simulink model "fboard_dwgn"  (Simulink 6.2)
settings: Solver=FixedStepDiscrete  SolverMode=SingleTasking  StartTime=0.0  StopTime=10.0  FixedStep=1  RelTol=1e-3
undefined symbols (not defined in the file): quant
libraries: xbsIndex_r3 x212, fb_xaui x1
(part 1 of 2)
settings Model: LastModifiedBy=mdexter
settings DebuggingCC: SolverPrmCheckMsg=warning

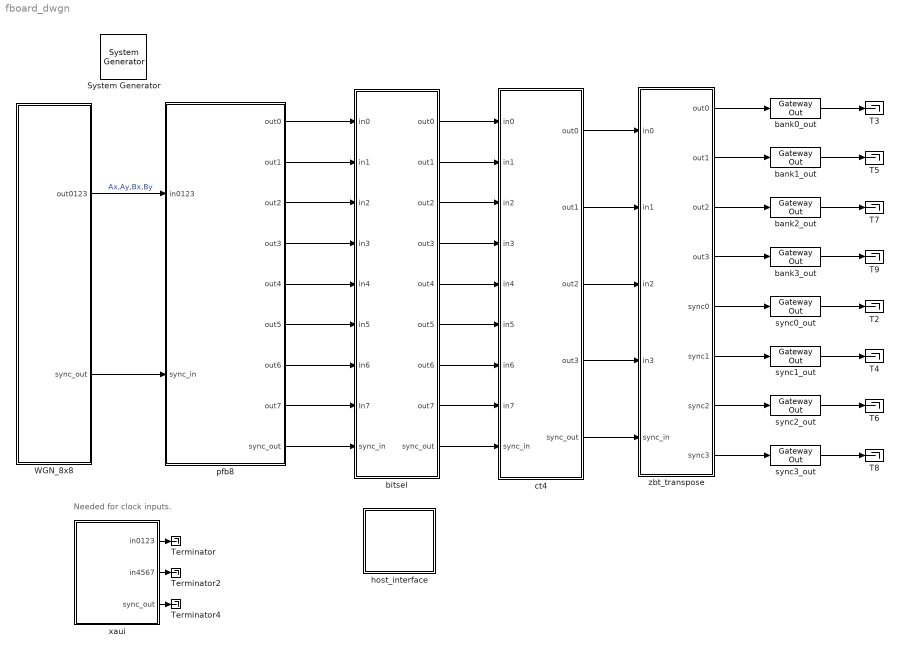
== system fboard_dwgn ==
  note: Needed for clock inputs.
  " System Generator" : xbsIndex_r3/ System Generator  Tag=genX  xilinxfamily=Virtex2P  part=xc2vp40  speed=-6  package=ff1152  synthesis_tool=XST  directory=./netlist  testbench=off  simulink_period=1  sysclk_period=100  incr_netlist=off  trim_vbits=Everywhere in SubSystem  dbl_ovrd=According to Block Masks  core_generation=According to Block Masks  run_coregen=off  deprecated_control=off  eval_field=0
      settings: AttributesFormatString=System\nGenerator
  T{2..9} (8 alike) : Terminator
  Terminator : Terminator
  Terminator2 : Terminator
  Terminator4 : Terminator
  WGN_8x8 : Subsystem
  bank0_out : xbsIndex_r3/Gateway Out  output_type=Double  nbits=8  bin_pt=6  arith_type=Boolean  quantization=Truncate  overflow=Wrap  hdl_port=on  timing_constraint=None  locs_specified=off  LOCs={}  needs_fixed_name=off  show_param=off
      settings: xl_area=[0, 0, 0, 0, 0, 0, 0]
  bank1_out : xbsIndex_r3/Gateway Out  output_type=Double  nbits=8  bin_pt=6  arith_type=Boolean  quantization=Truncate  overflow=Wrap  hdl_port=on  timing_constraint=None  locs_specified=off  LOCs={}  needs_fixed_name=off  show_param=off
      settings: xl_area=[0, 0, 0, 0, 0, 0, 0]
  bank2_out : xbsIndex_r3/Gateway Out  output_type=Double  nbits=8  bin_pt=6  arith_type=Boolean  quantization=Truncate  overflow=Wrap  hdl_port=on  timing_constraint=None  locs_specified=off  LOCs={}  needs_fixed_name=off  show_param=off
      settings: xl_area=[0, 0, 0, 0, 0, 0, 0]
  bank3_out : xbsIndex_r3/Gateway Out  output_type=Double  nbits=8  bin_pt=6  arith_type=Boolean  quantization=Truncate  overflow=Wrap  hdl_port=on  timing_constraint=None  locs_specified=off  LOCs={}  needs_fixed_name=off  show_param=off
      settings: xl_area=[0, 0, 0, 0, 0, 0, 0]
  bitsel : Subsystem
  ct4 : Subsystem
  host_interface : Subsystem
  pfb8 : Subsystem
  sync0_out : xbsIndex_r3/Gateway Out  output_type=Double  nbits=8  bin_pt=6  arith_type=Boolean  quantization=Truncate  overflow=Wrap  hdl_port=on  timing_constraint=None  locs_specified=off  LOCs={}  needs_fixed_name=off  show_param=off
      settings: xl_area=[0, 0, 0, 0, 0, 0, 0]
  sync1_out : xbsIndex_r3/Gateway Out  output_type=Double  nbits=8  bin_pt=6  arith_type=Boolean  quantization=Truncate  overflow=Wrap  hdl_port=on  timing_constraint=None  locs_specified=off  LOCs={}  needs_fixed_name=off  show_param=off
      settings: xl_area=[0, 0, 0, 0, 0, 0, 0]
  sync2_out : xbsIndex_r3/Gateway Out  output_type=Double  nbits=8  bin_pt=6  arith_type=Boolean  quantization=Truncate  overflow=Wrap  hdl_port=on  timing_constraint=None  locs_specified=off  LOCs={}  needs_fixed_name=off  show_param=off
      settings: xl_area=[0, 0, 0, 0, 0, 0, 0]
  sync3_out : xbsIndex_r3/Gateway Out  output_type=Double  nbits=8  bin_pt=6  arith_type=Boolean  quantization=Truncate  overflow=Wrap  hdl_port=on  timing_constraint=None  locs_specified=off  LOCs={}  needs_fixed_name=off  show_param=off
      settings: xl_area=[0, 0, 0, 0, 0, 0, 0]
  xaui : Subsystem
  zbt_transpose : Subsystem
  wires:
  WGN_8x8/1(out0123) -> pfb8/1(in0123)  "Ax,Ay,Bx,By"
  WGN_8x8/2(sync_out) -> pfb8/2(sync_in)
  sync0_out/1 -> T2/1
  bank0_out/1 -> T3/1
  sync1_out/1 -> T4/1
  bank1_out/1 -> T5/1
  sync2_out/1 -> T6/1
  bank2_out/1 -> T7/1
  sync3_out/1 -> T8/1
  bank3_out/1 -> T9/1
  pfb8/1(out0) -> bitsel/1(in0)
  pfb8/2(out1) -> bitsel/2(in1)
  pfb8/3(out2) -> bitsel/3(in2)
  pfb8/4(out3) -> bitsel/4(in3)
  pfb8/5(out4) -> bitsel/5(in4)
  pfb8/6(out5) -> bitsel/6(in5)
  pfb8/7(out6) -> bitsel/7(In6)
  pfb8/8(out7) -> bitsel/8(In7)
  pfb8/9(sync_out) -> bitsel/9(sync_in)
  bitsel/1(out0) -> ct4/1(in0)
  ct4/1(out0) -> zbt_transpose/1("in0\t")
  ct4/2(out1) -> zbt_transpose/2(in1)
  ct4/3(out2) -> zbt_transpose/3(in2)
  ct4/4(out3) -> zbt_transpose/4(in3)
  ct4/5(sync_out) -> zbt_transpose/5(sync_in)
  zbt_transpose/1(out0) -> bank0_out/1
  zbt_transpose/2(out1) -> bank1_out/1
  zbt_transpose/3(out2) -> bank2_out/1
  zbt_transpose/4(out3) -> bank3_out/1
  zbt_transpose/5(sync0) -> sync0_out/1
  zbt_transpose/6(sync1) -> sync1_out/1
  zbt_transpose/7(sync2) -> sync2_out/1
  zbt_transpose/8(sync3) -> sync3_out/1
  bitsel/2(out1) -> ct4/2(in1)
  bitsel/3(out2) -> ct4/3(in2)
  bitsel/4(out3) -> ct4/4(in3)
  bitsel/5(out4) -> ct4/5(in4)
  bitsel/6(out5) -> ct4/6(in5)
  bitsel/7(out6) -> ct4/7(in6)
  bitsel/8(out7) -> ct4/8(in7)
  bitsel/9(sync_out) -> ct4/9(sync_in)
  xaui/1(in0123) -> Terminator/1
  xaui/2(in4567) -> Terminator2/1
  xaui/3(sync_out) -> Terminator4/1

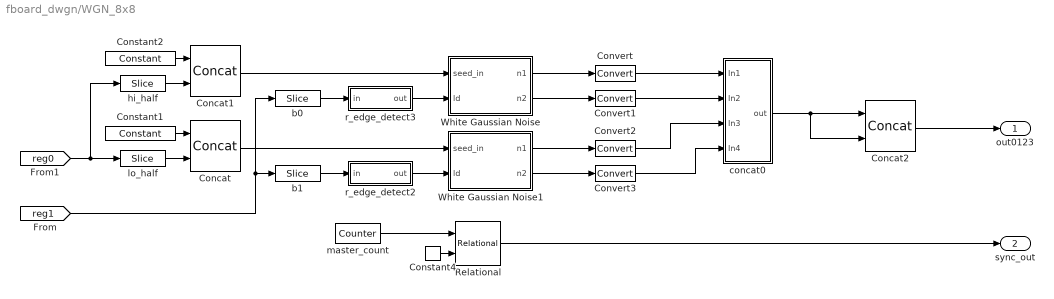
== system fboard_dwgn/WGN_8x8 ==
  Concat : xbsIndex_r3/Concat  num_inputs=2  explicit_period=off  period=1  dbl_ovrd=off
  Concat1 : xbsIndex_r3/Concat  num_inputs=2  explicit_period=off  period=1  dbl_ovrd=off
  Concat2 : xbsIndex_r3/Concat  num_inputs=2  explicit_period=off  period=1  dbl_ovrd=off
  Constant1 : xbsIndex_r3/Constant  const=hex2dec('bafd')  equ=P=C  arith_type=Unsigned  n_bits=16  bin_pt=0  opselect=C  inp2=PCIN>>17  opr=+  inp1=P  carry=CIN  iostate=0  explicit_period=on  period=1  dbl_ovrd=off
  Constant2 : xbsIndex_r3/Constant  const=hex2dec('bafd')  equ=P=C  arith_type=Unsigned  n_bits=16  bin_pt=0  opselect=C  inp2=PCIN>>17  opr=+  inp1=P  carry=CIN  iostate=0  explicit_period=on  period=1  dbl_ovrd=off
  Constant4 : xbsIndex_r3/Constant  const=0  equ=P=C  arith_type=Unsigned  n_bits=27  bin_pt=0  opselect=C  inp2=PCIN>>17  opr=+  inp1=P  carry=CIN  iostate=0  explicit_period=on  period=1  dbl_ovrd=off
  Convert{,1..3} (4 alike) : xbsIndex_r3/Convert  arith_type="Signed  (2's comp)"  n_bits=8  bin_pt=5  quantization="Round  (unbiased: +/- Inf)"  overflow=Wrap  latency=3  explicit_period=off  period=1  dbl_ovrd=off  show_param=on  inserted_by_tool=off  pipeline=on
      settings: xl_area=[0, 0, 0, 0, 0, 0, 0]
  Relational : xbsIndex_r3/Relational  mode=a=b  latency=1  explicit_period=off  period=1  en=off  dbl_ovrd=off  show_param=off
      settings: xl_area=[0, 0, 0, 0, 0, 0, 0]
  White Gaussian Noise : Subsystem  mask(Mask Type Goes Here){seed=hex2dec('12345678')}
      mask help: Mask Description Goes Here
      mask Help: Mask Help Goes Here
      mask CallbackString:
      | if str2num(get_param(gcb, 'seed')) == 0
      |     error('Seed cannot be zero.')
      | end
      mask Display:
      | port_label('input',1,'seed_in');
      | port_label('input',2,'ld');
      | port_label('output',1,'n1');
      | port_label('output',2,'n2');
  White Gaussian Noise1 : Subsystem  mask(Mask Type Goes Here){seed=hex2dec('12345678')}
      mask help: Mask Description Goes Here
      mask Help: Mask Help Goes Here
      mask CallbackString:
      | if str2num(get_param(gcb, 'seed')) == 0
      |     error('Seed cannot be zero.')
      | end
      mask Display:
      | port_label('input',1,'seed_in');
      | port_label('input',2,'ld');
      | port_label('output',1,'n1');
      | port_label('output',2,'n2');
  b0 : xbsIndex_r3/Slice  mode=Lower Bit Location + Width  nbits=1  bit1=0  base1=MSB of Input  bit0=0  base0=LSB of Input  boolean_output=on  explicit_period=off  period=1  dbl_ovrd=off
  b1 : xbsIndex_r3/Slice  mode=Lower Bit Location + Width  nbits=1  bit1=0  base1=MSB of Input  bit0=1  base0=LSB of Input  boolean_output=on  explicit_period=off  period=1  dbl_ovrd=off
  concat0 : Subsystem
  hi_half : xbsIndex_r3/Slice  mode=Upper Bit Location + Width  nbits=16  bit1=0  base1=MSB of Input  bit0=0  base0=LSB of Input  boolean_output=off  explicit_period=off  period=1  dbl_ovrd=off
  lo_half : xbsIndex_r3/Slice  mode=Lower Bit Location + Width  nbits=16  bit1=0  base1=MSB of Input  bit0=0  base0=LSB of Input  boolean_output=off  explicit_period=off  period=1  dbl_ovrd=off
  master_count : xbsIndex_r3/Counter  cnt_type=Free Running  n_bits=27  bin_pt=0  arith_type=Unsigned  start_count=0  cnt_to=Inf  cnt_by_val=1  operation=Up  explicit_period=off  period=1  load_pin=off  rst=off  en=off  dbl_ovrd=off  show_param=on  use_rpm=on  gen_core=off
      settings: xl_area=[0, 0, 0, 0, 0, 0, 0]
  r_edge_detect2 : Subsystem
  r_edge_detect3 : Subsystem
  out0123 : Outport
  sync_out : Outport  Port=2
  wires:
  White Gaussian Noise/1(n1) -> Convert/1
  White Gaussian Noise/2(n2) -> Convert1/1
  White Gaussian Noise1/1(n1) -> Convert2/1
  White Gaussian Noise1/2(n2) -> Convert3/1
  Convert/1 -> concat0/1(In1)
  Convert1/1 -> concat0/2(In2)
  Convert2/1 -> concat0/3(In3)
  Convert3/1 -> concat0/4(In4)
  concat0/1(out) -> Concat2/1, Concat2/2
  [reg1] -> b0/1, b1/1
  b0/1 -> r_edge_detect3/1(in)
  b1/1 -> r_edge_detect2/1(in)
  r_edge_detect2/1(out) -> White Gaussian Noise1/2(ld)
  r_edge_detect3/1(out) -> White Gaussian Noise/2(ld)
  master_count/1 -> Relational/1
  lo_half/1 -> Concat/2
  hi_half/1 -> Concat1/2
  Relational/1 -> sync_out/1
  [reg0] -> lo_half/1, hi_half/1
  Concat1/1 -> White Gaussian Noise/1(seed_in)
  Concat/1 -> White Gaussian Noise1/1(seed_in)
  Constant1/1 -> Concat/1
  Constant2/1 -> Concat1/1
  Constant4/1 -> Relational/2
  Concat2/1 -> out0123/1

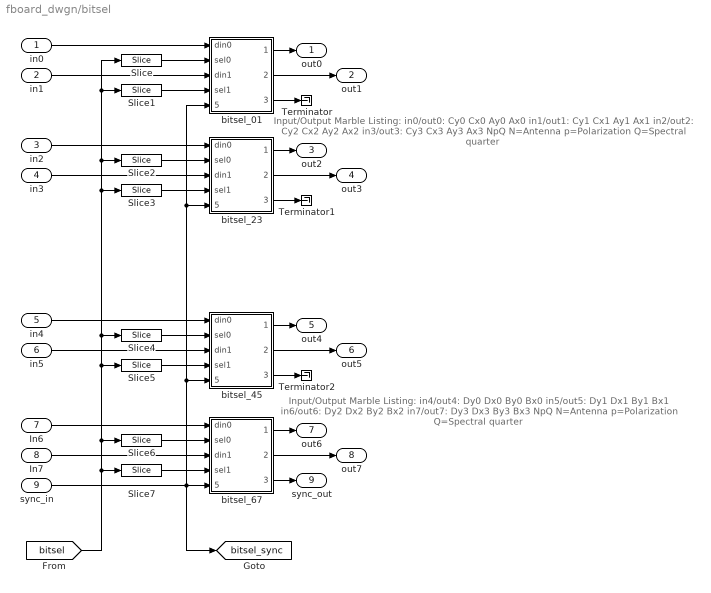
== system fboard_dwgn/bitsel ==
  note: Input/Output Marble Listing:
      |
      | in0/out0: Cy0 Cx0 Ay0 Ax0
      | in1/out1: Cy1 Cx1 Ay1 Ax1
      | in2/out2: Cy2 Cx2 Ay2 Ax2
      | in3/out3: Cy3 Cx3 Ay3 Ax3
      |
      | NpQ
      | N=Antenna
      | p=Polarization
      | Q=Spectral quarter
  note: Input/Output Marble Listing:
      |
      | in4/out4: Dy0 Dx0 By0 Bx0
      | in5/out5: Dy1 Dx1 By1 Bx1
      | in6/out6: Dy2 Dx2 By2 Bx2
      | in7/out7: Dy3 Dx3 By3 Bx3
      |
      | NpQ
      | N=Antenna
      | p=Polarization
      | Q=Spectral quarter
  in0 : Inport  Port=1  LatchInput=off
  in1 : Inport  Port=2  LatchInput=off
  in2 : Inport  Port=3  LatchInput=off
  in3 : Inport  Port=4  LatchInput=off
  in4 : Inport  Port=5  LatchInput=off
  in5 : Inport  Port=6  LatchInput=off
  In6 : Inport  Port=7  LatchInput=off
  In7 : Inport  Port=8  LatchInput=off
  sync_in : Inport  Port=9  LatchInput=off
  Slice : xbsIndex_r3/Slice  mode=Lower Bit Location + Width  nbits=4  bit1=0  base1=MSB of Input  bit0=0  base0=LSB of Input  boolean_output=off  explicit_period=off  period=1  dbl_ovrd=off
  Slice1 : xbsIndex_r3/Slice  mode=Lower Bit Location + Width  nbits=4  bit1=0  base1=MSB of Input  bit0=4  base0=LSB of Input  boolean_output=off  explicit_period=off  period=1  dbl_ovrd=off
  Slice2 : xbsIndex_r3/Slice  mode=Lower Bit Location + Width  nbits=4  bit1=0  base1=MSB of Input  bit0=8  base0=LSB of Input  boolean_output=off  explicit_period=off  period=1  dbl_ovrd=off
  Slice3 : xbsIndex_r3/Slice  mode=Lower Bit Location + Width  nbits=4  bit1=0  base1=MSB of Input  bit0=12  base0=LSB of Input  boolean_output=off  explicit_period=off  period=1  dbl_ovrd=off
  Slice4 : xbsIndex_r3/Slice  mode=Lower Bit Location + Width  nbits=4  bit1=0  base1=MSB of Input  bit0=16  base0=LSB of Input  boolean_output=off  explicit_period=off  period=1  dbl_ovrd=off
  Slice5 : xbsIndex_r3/Slice  mode=Lower Bit Location + Width  nbits=4  bit1=0  base1=MSB of Input  bit0=20  base0=LSB of Input  boolean_output=off  explicit_period=off  period=1  dbl_ovrd=off
  Slice6 : xbsIndex_r3/Slice  mode=Lower Bit Location + Width  nbits=4  bit1=0  base1=MSB of Input  bit0=24  base0=LSB of Input  boolean_output=off  explicit_period=off  period=1  dbl_ovrd=off
  Slice7 : xbsIndex_r3/Slice  mode=Lower Bit Location + Width  nbits=4  bit1=0  base1=MSB of Input  bit0=28  base0=LSB of Input  boolean_output=off  explicit_period=off  period=1  dbl_ovrd=off
  Terminator : Terminator
  Terminator1 : Terminator
  Terminator2 : Terminator
  bitsel_01 : Subsystem
  bitsel_23 : Subsystem
  bitsel_45 : Subsystem
  bitsel_67 : Subsystem
  out0 : Outport
  out1 : Outport  Port=2
  out2 : Outport  Port=3
  out3 : Outport  Port=4
  out4 : Outport  Port=5
  out5 : Outport  Port=6
  out6 : Outport  Port=7
  out7 : Outport  Port=8
  sync_out : Outport  Port=9
  tag scope: bitsel_sync=global
  wires:
  in0/1 -> bitsel_01/1(din0)
  bitsel_01/1(dout0) -> out0/1
  in1/1 -> bitsel_01/3(din1)
  in2/1 -> bitsel_23/1(din0)
  in3/1 -> bitsel_23/3(din1)
  in4/1 -> bitsel_45/1(din0)
  in5/1 -> bitsel_45/3(din1)
  In6/1 -> bitsel_67/1(din0)
  In7/1 -> bitsel_67/3(din1)
  sync_in/1 -> [bitsel_sync], bitsel_01/5(sync_in), bitsel_23/5(sync_in), bitsel_45/5(sync_in), bitsel_67/5(sync_in)
  Slice/1 -> bitsel_01/2(sel0)
  Slice1/1 -> bitsel_01/4(sel1)
  Slice2/1 -> bitsel_23/2(sel0)
  Slice3/1 -> bitsel_23/4(sel1)
  Slice4/1 -> bitsel_45/2(sel0)
  Slice5/1 -> bitsel_45/4(sel1)
  Slice6/1 -> bitsel_67/2(sel0)
  Slice7/1 -> bitsel_67/4(sel1)
  [bitsel] -> Slice5/1, Slice4/1, Slice3/1, Slice2/1, Slice1/1, Slice/1, Slice6/1, Slice7/1
  bitsel_01/3(sync_out) -> Terminator/1
  bitsel_01/2(dout1) -> out1/1
  bitsel_23/1(dout0) -> out2/1
  bitsel_23/3(sync_out) -> Terminator1/1
  bitsel_23/2(dout1) -> out3/1
  bitsel_45/1(dout0) -> out4/1
  bitsel_45/3(sync_out) -> Terminator2/1
  bitsel_45/2(dout1) -> out5/1
  bitsel_67/1(dout0) -> out6/1
  bitsel_67/2(dout1) -> out7/1
  bitsel_67/3(sync_out) -> sync_out/1

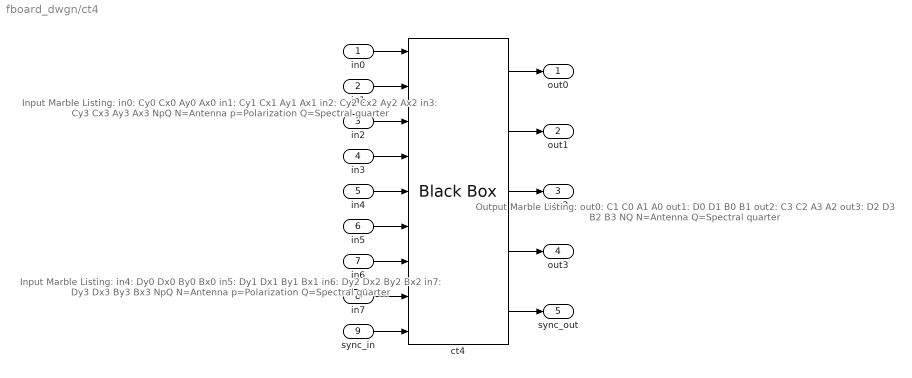
== system fboard_dwgn/ct4 ==
  note: Input Marble Listing:
      |
      | in0: Cy0 Cx0 Ay0 Ax0
      | in1: Cy1 Cx1 Ay1 Ax1
      | in2: Cy2 Cx2 Ay2 Ax2
      | in3: Cy3 Cx3 Ay3 Ax3
      |
      | NpQ
      | N=Antenna
      | p=Polarization
      | Q=Spectral quarter
  note: Input Marble Listing:
      |
      | in4: Dy0 Dx0 By0 Bx0
      | in5: Dy1 Dx1 By1 Bx1
      | in6: Dy2 Dx2 By2 Bx2
      | in7: Dy3 Dx3 By3 Bx3
      |
      | NpQ
      | N=Antenna
      | p=Polarization
      | Q=Spectral quarter
  note: Output Marble Listing:
      |
      | out0: C1 C0 A1 A0
      | out1: D0 D1 B0 B1
      | out2: C3 C2 A3 A2
      | out3: D2 D3 B2 B3
      |
      | NQ
      | N=Antenna
      | Q=Spectral quarter
  in0 : Inport  Port=1  LatchInput=off
  in1 : Inport  Port=2  LatchInput=off
  in2 : Inport  Port=3  LatchInput=off
  in3 : Inport  Port=4  LatchInput=off
  in4 : Inport  Port=5  LatchInput=off
  in5 : Inport  Port=6  LatchInput=off
  in6 : Inport  Port=7  LatchInput=off
  in7 : Inport  Port=8  LatchInput=off
  sync_in : Inport  Port=9  LatchInput=off
  ct4 : xbsIndex_r3/Black Box  init_code=ct4_config  sim_method=Inactive  show_param=off
      settings: xl_area=[0, 0, 0, 0, 0, 0, 0]
  out0 : Outport
  out1 : Outport  Port=2
  out2 : Outport  Port=3
  out3 : Outport  Port=4
  sync_out : Outport  Port=5
  wires:
  in0/1 -> ct4/1
  ct4/1 -> out0/1
  in1/1 -> ct4/2
  ct4/2 -> out1/1
  in2/1 -> ct4/3
  ct4/3 -> out2/1
  in3/1 -> ct4/4
  ct4/4 -> out3/1
  in4/1 -> ct4/5
  ct4/5 -> sync_out/1
  in5/1 -> ct4/6
  in6/1 -> ct4/7
  in7/1 -> ct4/8
  sync_in/1 -> ct4/9

== system fboard_dwgn/host_interface ==
  Constant2 : xbsIndex_r3/Constant  const=hex2dec('baff7ed')  equ=P=C  arith_type=Unsigned  n_bits=32  bin_pt=0  opselect=C  inp2=PCIN>>17  opr=+  inp1=P  carry=CIN  iostate=0  explicit_period=on  period=1  dbl_ovrd=off
  T12 : Terminator
  host_interface : xbsIndex_r3/Black Box  init_code=host_interface_config  sim_method=Inactive  show_param=off
      settings: xl_area=[0, 0, 0, 0, 0, 0, 0]
  reset : xbsIndex_r3/Gateway Out  output_type=Double  nbits=8  bin_pt=6  arith_type=Boolean  quantization=Truncate  overflow=Wrap  hdl_port=on  timing_constraint=None  locs_specified=off  LOCs={}  needs_fixed_name=off  show_param=off
      settings: xl_area=[0, 0, 0, 0, 0, 0, 0]
  tag scope: bitsel=global, reg0=global, reg1=global, reset=global
  wires:
  reset/1 -> T12/1
  [bitsel_sync] -> host_interface/1
  host_interface/4 -> reset/1, [reset]
  host_interface/1 -> [bitsel]
  host_interface/2 -> [reg0]
  host_interface/3 -> [reg1]
  Constant2/1 -> host_interface/2, host_interface/3, host_interface/4, host_interface/5, host_interface/6, host_interface/7, host_interface/8

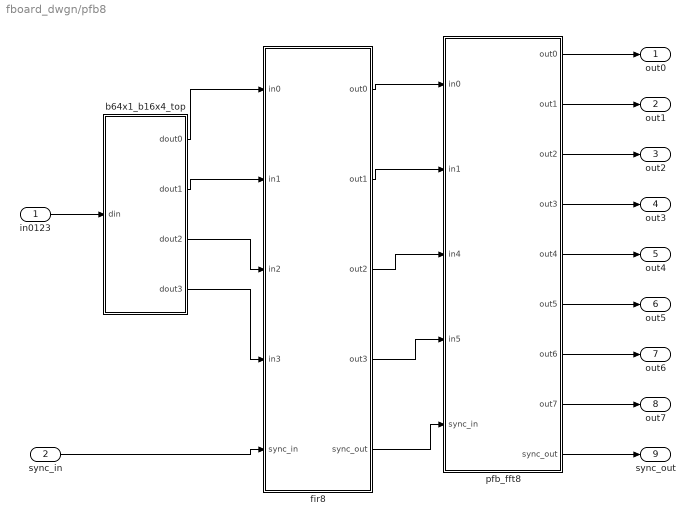
== system fboard_dwgn/pfb8 ==
  in0123 : Inport  Port=1  LatchInput=off
  sync_in : Inport  Port=2  LatchInput=off
  b64x1_b16x4_top : Subsystem
  fir8 : Subsystem  mask{fb_ntaps=4}
      mask prompts: fb_ntaps "Number of taps"
  pfb_fft8 : Subsystem
  out0 : Outport
  out1 : Outport  Port=2
  out2 : Outport  Port=3
  out3 : Outport  Port=4
  out4 : Outport  Port=5
  out5 : Outport  Port=6
  out6 : Outport  Port=7
  out7 : Outport  Port=8
  sync_out : Outport  Port=9
  wires:
  fir8/5(sync_out) -> pfb_fft8/5(sync_in)
  fir8/2(out1) -> pfb_fft8/2(in1)
  fir8/1(out0) -> pfb_fft8/1(in0)
  b64x1_b16x4_top/2(dout1) -> fir8/2(in1)
  b64x1_b16x4_top/1(dout0) -> fir8/1(in0)
  b64x1_b16x4_top/4(dout3) -> fir8/4(in3)
  b64x1_b16x4_top/3(dout2) -> fir8/3(in2)
  pfb_fft8/1(out0) -> out0/1
  pfb_fft8/2(out1) -> out1/1
  in0123/1 -> b64x1_b16x4_top/1(din)
  pfb_fft8/3(out2) -> out2/1
  pfb_fft8/4(out3) -> out3/1
  pfb_fft8/5(out4) -> out4/1
  pfb_fft8/6(out5) -> out5/1
  pfb_fft8/7(out6) -> out6/1
  pfb_fft8/8(out7) -> out7/1
  pfb_fft8/9(sync_out) -> sync_out/1
  sync_in/1 -> fir8/5(sync_in)
  fir8/3(out2) -> pfb_fft8/3(in4)
  fir8/4(out3) -> pfb_fft8/4(in5)

== system fboard_dwgn/xaui ==
  Constant : xbsIndex_r3/Constant  const=0  equ=P=C  arith_type=Boolean  n_bits=1  bin_pt=0  opselect=C  inp2=PCIN>>17  opr=+  inp1=P  carry=CIN  iostate=0  explicit_period=on  period=1  dbl_ovrd=off
  Constant1 : xbsIndex_r3/Constant  const=1  equ=P=C  arith_type=Boolean  n_bits=1  bin_pt=0  opselect=C  inp2=PCIN>>17  opr=+  inp1=P  carry=CIN  iostate=0  explicit_period=on  period=1  dbl_ovrd=off
  Slice : xbsIndex_r3/Slice  mode=Lower Bit Location + Width  nbits=1  bit1=0  base1=MSB of Input  bit0=0  base0=LSB of Input  boolean_output=on  explicit_period=off  period=1  dbl_ovrd=off
  Slice1 : xbsIndex_r3/Slice  mode=Lower Bit Location + Width  nbits=1  bit1=0  base1=MSB of Input  bit0=0  base0=LSB of Input  boolean_output=on  explicit_period=off  period=1  dbl_ovrd=off
  fb_xaui : fb_xaui/fb_xaui
  realign : Subsystem
  status_monitor : Subsystem
  sync_monitor : Subsystem
  sync_sel : Subsystem
  in0123 : Outport
  in4567 : Outport  Port=2
  sync_out : Outport  Port=3
  wires:
  Constant/1 -> fb_xaui/1
  Constant1/1 -> fb_xaui/2
  fb_xaui/6 -> status_monitor/2(bot_status)
  fb_xaui/3 -> status_monitor/1(top_status)
  fb_xaui/1 -> realign/1(din0)
  fb_xaui/2 -> Slice/1
  fb_xaui/4 -> realign/3(din1)
  fb_xaui/5 -> Slice1/1
  Slice/1 -> sync_monitor/1(top_sync), realign/2(sync0), sync_sel/1(top_sync)
  Slice1/1 -> sync_monitor/2(bot_sync), realign/4(sync1), sync_sel/2(bot_sync)
  realign/1(dout0) -> in0123/1
  realign/2(dout1) -> in4567/1
  realign/3(sync_out) -> sync_out/1
  sync_sel/1(sync_out) -> realign/5(sync_in)

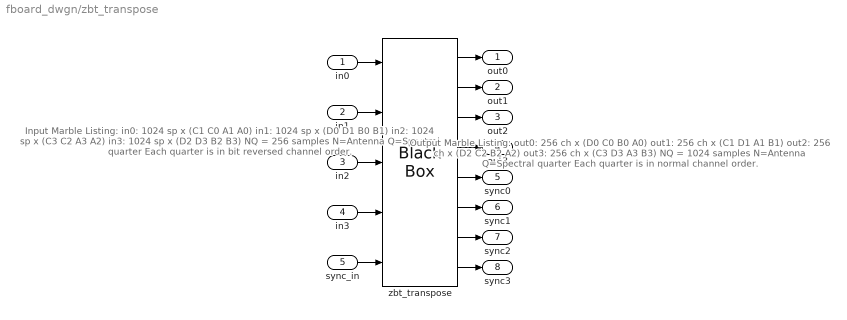
== system fboard_dwgn/zbt_transpose ==
  note: Input Marble Listing:
      |
      | in0: 1024 sp x (C1 C0 A1 A0)
      | in1: 1024 sp x (D0 D1 B0 B1)
      | in2: 1024 sp x (C3 C2 A3 A2)
      | in3: 1024 sp x (D2 D3 B2 B3)
      |
      | NQ = 256 samples
      |
      | N=Antenna
      | Q=Spectral quarter
      |
      | Each quarter is in bit
      | reversed channel order.
  note: Output Marble Listing:
      |
      | out0: 256 ch x (D0 C0 B0 A0)
      | out1: 256 ch x (C1 D1 A1 B1)
      | out2: 256 ch x (D2 C2 B2 A2)
      | out3: 256 ch x (C3 D3 A3 B3)
      |
      | NQ = 1024 samples
      |
      | N=Antenna
      | Q=Spectral quarter
      |
      | Each quarter is in
      | normal channel order.
  "in0\t" : Inport  Port=1  LatchInput=off
  in1 : Inport  Port=2  LatchInput=off
  in2 : Inport  Port=3  LatchInput=off
  in3 : Inport  Port=4  LatchInput=off
  sync_in : Inport  Port=5  LatchInput=off
  zbt_transpose : xbsIndex_r3/Black Box  init_code=zbt_transpose_config  sim_method=Inactive  show_param=off
      settings: xl_area=[0, 0, 0, 0, 0, 0, 0]
  out0 : Outport
  out1 : Outport  Port=2
  out2 : Outport  Port=3
  out3 : Outport  Port=4
  sync0 : Outport  Port=5
  sync1 : Outport  Port=6
  sync2 : Outport  Port=7
  sync3 : Outport  Port=8
  wires:
  zbt_transpose/1 -> out0/1
  "in0\t"/1 -> zbt_transpose/1
  zbt_transpose/2 -> out1/1
  in1/1 -> zbt_transpose/2
  zbt_transpose/3 -> out2/1
  zbt_transpose/4 -> out3/1
  in2/1 -> zbt_transpose/3
  zbt_transpose/5 -> sync0/1
  in3/1 -> zbt_transpose/4
  zbt_transpose/6 -> sync1/1
  zbt_transpose/7 -> sync2/1
  sync_in/1 -> zbt_transpose/5
  zbt_transpose/8 -> sync3/1

== system fboard_dwgn/WGN_8x8/White Gaussian Noise ==
  seed_in : Inport  Port=1  LatchInput=off
  ld : Inport  Port=2  LatchInput=off
  tt800_prng : Subsystem
  tt800_seed_gen : Subsystem
  u2n : Subsystem
  n1 : Outport
  n2 : Outport  Port=2
  wires:
  tt800_prng/1(out) -> u2n/1(u)
  tt800_seed_gen/1(seed_out) -> tt800_prng/1(seed)
  tt800_seed_gen/2(seed_en) -> tt800_prng/2(seed_en)
  seed_in/1 -> tt800_seed_gen/1(seed_in)
  u2n/1(n1) -> n1/1
  ld/1 -> tt800_seed_gen/2(ld)
  u2n/2(n2) -> n2/1

== system fboard_dwgn/WGN_8x8/White Gaussian Noise1 ==
  seed_in : Inport  Port=1  LatchInput=off
  ld : Inport  Port=2  LatchInput=off
  tt800_prng : Subsystem
  tt800_seed_gen : Subsystem
  u2n : Subsystem
  n1 : Outport
  n2 : Outport  Port=2
  wires:
  tt800_prng/1(out) -> u2n/1(u)
  tt800_seed_gen/1(seed_out) -> tt800_prng/1(seed)
  tt800_seed_gen/2(seed_en) -> tt800_prng/2(seed_en)
  seed_in/1 -> tt800_seed_gen/1(seed_in)
  u2n/1(n1) -> n1/1
  ld/1 -> tt800_seed_gen/2(ld)
  u2n/2(n2) -> n2/1

== system fboard_dwgn/WGN_8x8/concat0 ==
  In1 : Inport  Port=1  LatchInput=off
  In2 : Inport  Port=2  LatchInput=off
  In3 : Inport  Port=3  LatchInput=off
  In4 : Inport  Port=4  LatchInput=off
  ri_to_c : Subsystem  mask(Real-Imag to Complex){}
      mask help: Concatenates real and imaginary inputs into a complex output.
      mask init:
      | ri_to_c_init(gcb);
      mask Help:
      | <pre>
      | Description::
      | 
      | Concatenates a real and imaginary input into a complex output.
      | Useful for simplifying interconnects.
      | See also: Complex to Real-Imag (c_to_ri)
      | 
      | Mask Parameters::
      | 
      | (N/A)
      | </pre>
  ri_to_c1 : Subsystem  mask(Real-Imag to Complex){}
      mask help: Concatenates real and imaginary inputs into a complex output.
      mask init:
      | ri_to_c_init(gcb);
      mask Help:
      | <pre>
      | Description::
      | 
      | Concatenates a real and imaginary input into a complex output.
      | Useful for simplifying interconnects.
      | See also: Complex to Real-Imag (c_to_ri)
      | 
      | Mask Parameters::
      | 
      | (N/A)
      | </pre>
  ri_to_c2 : Subsystem  mask(Real-Imag to Complex){}
      mask help: Concatenates real and imaginary inputs into a complex output.
      mask init:
      | ri_to_c_init(gcb);
      mask Help:
      | <pre>
      | Description::
      | 
      | Concatenates a real and imaginary input into a complex output.
      | Useful for simplifying interconnects.
      | See also: Complex to Real-Imag (c_to_ri)
      | 
      | Mask Parameters::
      | 
      | (N/A)
      | </pre>
  out : Outport
  wires:
  ri_to_c/1(c) -> ri_to_c2/1(re)
  ri_to_c1/1(c) -> ri_to_c2/2(im)
  In1/1 -> ri_to_c/1(re)
  In2/1 -> ri_to_c/2(im)
  ri_to_c2/1(c) -> out/1
  In3/1 -> ri_to_c1/1(re)
  In4/1 -> ri_to_c1/2(im)

== system fboard_dwgn/WGN_8x8/r_edge_detect2 ==
  in : Inport  Port=1  LatchInput=off
  Delay : xbsIndex_r3/Delay  latency=1  reg_retiming=off  explicit_period=off  period=1  en=off  accept_only_valid=off  init_zero=on  dbl_ovrd=off  show_param=off
      settings: xl_area=[1 1 0 0 0 0 0]
  Expression : xbsIndex_r3/Expression  expression=curr & ~prev  precision=Full  arith_type=Unsigned  n_bits=8  bin_pt=2  align_bp=on  latency=0  explicit_period=off  period=1  en=off  dbl_ovrd=off  show_param=off
      settings: xl_area=[0, 0, 0, 0, 0, 0, 0]
  out : Outport
  wires:
  in/1 -> Expression/1, Delay/1
  Delay/1 -> Expression/2
  Expression/1 -> out/1

== system fboard_dwgn/WGN_8x8/r_edge_detect3 ==
  in : Inport  Port=1  LatchInput=off
  Delay : xbsIndex_r3/Delay  latency=1  reg_retiming=off  explicit_period=off  period=1  en=off  accept_only_valid=off  init_zero=on  dbl_ovrd=off  show_param=off
      settings: xl_area=[1 1 0 0 0 0 0]
  Expression : xbsIndex_r3/Expression  expression=curr & ~prev  precision=Full  arith_type=Unsigned  n_bits=8  bin_pt=2  align_bp=on  latency=0  explicit_period=off  period=1  en=off  dbl_ovrd=off  show_param=off
      settings: xl_area=[0, 0, 0, 0, 0, 0, 0]
  out : Outport
  wires:
  Expression/1 -> out/1
  Delay/1 -> Expression/2
  in/1 -> Delay/1, Expression/1

== system fboard_dwgn/bitsel/bitsel_01 ==
  note: If bitsel black box is too expensive,
      | use fixed bit selection via
      | complex_convert with 19_8 in.
  din0 : Inport  Port=1  LatchInput=off
  sel0 : Inport  Port=2  LatchInput=off
  din1 : Inport  Port=3  LatchInput=off
  sel1 : Inport  Port=4  LatchInput=off
  sync_in : Inport  Port=5  LatchInput=off
  Constant : xbsIndex_r3/Constant  const=0  equ=P=C  arith_type=Boolean  n_bits=1  bin_pt=0  opselect=C  inp2=PCIN>>17  opr=+  inp1=P  carry=CIN  iostate=0  explicit_period=on  period=1  dbl_ovrd=off
  Terminator : Terminator
  bitsel_0 : xbsIndex_r3/Black Box  init_code=bitsel_config  sim_method=Inactive  show_param=off
      settings: xl_area=[0, 0, 0, 0, 0, 0, 0]
  bitsel_1 : xbsIndex_r3/Black Box  init_code=bitsel_config  sim_method=Inactive  show_param=off
      settings: xl_area=[0, 0, 0, 0, 0, 0, 0]
  dout0 : Outport
  dout1 : Outport  Port=2
  sync_out : Outport  Port=3
  wires:
  din0/1 -> bitsel_0/1
  din1/1 -> bitsel_1/1
  sel0/1 -> bitsel_0/2
  bitsel_0/1 -> dout0/1
  sel1/1 -> bitsel_1/2
  bitsel_1/1 -> dout1/1
  sync_in/1 -> bitsel_1/3
  bitsel_1/2 -> sync_out/1
  Constant/1 -> bitsel_0/3
  bitsel_0/2 -> Terminator/1

== system fboard_dwgn/bitsel/bitsel_23 ==
  note: If bitsel black box is too expensive,
      | use fixed bit selection via
      | complex_convert with 19_8 in.
  din0 : Inport  Port=1  LatchInput=off
  sel0 : Inport  Port=2  LatchInput=off
  din1 : Inport  Port=3  LatchInput=off
  sel1 : Inport  Port=4  LatchInput=off
  sync_in : Inport  Port=5  LatchInput=off
  Constant : xbsIndex_r3/Constant  const=0  equ=P=C  arith_type=Boolean  n_bits=1  bin_pt=0  opselect=C  inp2=PCIN>>17  opr=+  inp1=P  carry=CIN  iostate=0  explicit_period=on  period=1  dbl_ovrd=off
  Terminator : Terminator
  bitsel_0 : xbsIndex_r3/Black Box  init_code=bitsel_config  sim_method=Inactive  show_param=off
      settings: xl_area=[0, 0, 0, 0, 0, 0, 0]
  bitsel_1 : xbsIndex_r3/Black Box  init_code=bitsel_config  sim_method=Inactive  show_param=off
      settings: xl_area=[0, 0, 0, 0, 0, 0, 0]
  dout0 : Outport
  dout1 : Outport  Port=2
  sync_out : Outport  Port=3
  wires:
  bitsel_0/2 -> Terminator/1
  Constant/1 -> bitsel_0/3
  bitsel_1/2 -> sync_out/1
  sync_in/1 -> bitsel_1/3
  bitsel_1/1 -> dout1/1
  sel1/1 -> bitsel_1/2
  bitsel_0/1 -> dout0/1
  sel0/1 -> bitsel_0/2
  din1/1 -> bitsel_1/1
  din0/1 -> bitsel_0/1

== system fboard_dwgn/bitsel/bitsel_45 ==
  note: If bitsel black box is too expensive,
      | use fixed bit selection via
      | complex_convert with 19_8 in.
  din0 : Inport  Port=1  LatchInput=off
  sel0 : Inport  Port=2  LatchInput=off
  din1 : Inport  Port=3  LatchInput=off
  sel1 : Inport  Port=4  LatchInput=off
  sync_in : Inport  Port=5  LatchInput=off
  Constant : xbsIndex_r3/Constant  const=0  equ=P=C  arith_type=Boolean  n_bits=1  bin_pt=0  opselect=C  inp2=PCIN>>17  opr=+  inp1=P  carry=CIN  iostate=0  explicit_period=on  period=1  dbl_ovrd=off
  Terminator : Terminator
  bitsel_0 : xbsIndex_r3/Black Box  init_code=bitsel_config  sim_method=Inactive  show_param=off
      settings: xl_area=[0, 0, 0, 0, 0, 0, 0]
  bitsel_1 : xbsIndex_r3/Black Box  init_code=bitsel_config  sim_method=Inactive  show_param=off
      settings: xl_area=[0, 0, 0, 0, 0, 0, 0]
  dout0 : Outport
  dout1 : Outport  Port=2
  sync_out : Outport  Port=3
  wires:
  din0/1 -> bitsel_0/1
  din1/1 -> bitsel_1/1
  sel0/1 -> bitsel_0/2
  bitsel_0/1 -> dout0/1
  sel1/1 -> bitsel_1/2
  bitsel_1/1 -> dout1/1
  sync_in/1 -> bitsel_1/3
  bitsel_1/2 -> sync_out/1
  Constant/1 -> bitsel_0/3
  bitsel_0/2 -> Terminator/1

== system fboard_dwgn/bitsel/bitsel_67 ==
  note: If bitsel black box is too expensive,
      | use fixed bit selection via
      | complex_convert with 19_8 in.
  din0 : Inport  Port=1  LatchInput=off
  sel0 : Inport  Port=2  LatchInput=off
  din1 : Inport  Port=3  LatchInput=off
  sel1 : Inport  Port=4  LatchInput=off
  sync_in : Inport  Port=5  LatchInput=off
  Constant : xbsIndex_r3/Constant  const=0  equ=P=C  arith_type=Boolean  n_bits=1  bin_pt=0  opselect=C  inp2=PCIN>>17  opr=+  inp1=P  carry=CIN  iostate=0  explicit_period=on  period=1  dbl_ovrd=off
  Terminator : Terminator
  bitsel_0 : xbsIndex_r3/Black Box  init_code=bitsel_config  sim_method=Inactive  show_param=off
      settings: xl_area=[0, 0, 0, 0, 0, 0, 0]
  bitsel_1 : xbsIndex_r3/Black Box  init_code=bitsel_config  sim_method=Inactive  show_param=off
      settings: xl_area=[0, 0, 0, 0, 0, 0, 0]
  dout0 : Outport
  dout1 : Outport  Port=2
  sync_out : Outport  Port=3
  wires:
  bitsel_0/2 -> Terminator/1
  Constant/1 -> bitsel_0/3
  bitsel_1/2 -> sync_out/1
  sync_in/1 -> bitsel_1/3
  bitsel_1/1 -> dout1/1
  sel1/1 -> bitsel_1/2
  bitsel_0/1 -> dout0/1
  sel0/1 -> bitsel_0/2
  din1/1 -> bitsel_1/1
  din0/1 -> bitsel_0/1

== system fboard_dwgn/pfb8/b64x1_b16x4_top ==
  din : Inport  Port=1  LatchInput=off
  Slice0 : xbsIndex_r3/Slice  mode=Lower Bit Location + Width  nbits=16  bit1=0  base1=LSB of Input  bit0=0  base0=LSB of Input  boolean_output=off  explicit_period=off  period=1  dbl_ovrd=off
  Slice1 : xbsIndex_r3/Slice  mode=Lower Bit Location + Width  nbits=16  bit1=0  base1=LSB of Input  bit0=16  base0=LSB of Input  boolean_output=off  explicit_period=off  period=1  dbl_ovrd=off
  Slice2 : xbsIndex_r3/Slice  mode=Lower Bit Location + Width  nbits=16  bit1=0  base1=LSB of Input  bit0=32  base0=LSB of Input  boolean_output=off  explicit_period=off  period=1  dbl_ovrd=off
  Slice3 : xbsIndex_r3/Slice  mode=Lower Bit Location + Width  nbits=16  bit1=0  base1=LSB of Input  bit0=48  base0=LSB of Input  boolean_output=off  explicit_period=off  period=1  dbl_ovrd=off
  dout0 : Outport
  dout1 : Outport  Port=2
  dout2 : Outport  Port=3
  dout3 : Outport  Port=4
  wires:
  din/1 -> Slice3/1, Slice2/1, Slice0/1, Slice1/1
  Slice3/1 -> dout0/1
  Slice2/1 -> dout1/1
  Slice1/1 -> dout2/1
  Slice0/1 -> dout3/1

== system fboard_dwgn/pfb8/fir8 ==
  in0 : Inport  Port=1  LatchInput=off
  in1 : Inport  Port=2  LatchInput=off
  in2 : Inport  Port=3  LatchInput=off
  in3 : Inport  Port=4  LatchInput=off
  sync_in : Inport  Port=5  LatchInput=off
  Terminator : Terminator
  pfb_fir_0 : Subsystem
  pfb_fir_1 : Subsystem
  out0 : Outport
  out1 : Outport  Port=2
  out2 : Outport  Port=3
  out3 : Outport  Port=4
  sync_out : Outport  Port=5
  wires:
  in0/1 -> pfb_fir_0/1(pol1_in)
  pfb_fir_0/1(pol1_out) -> out0/1
  in1/1 -> pfb_fir_0/2(pol2_in)
  pfb_fir_0/2(pol2_out) -> out1/1
  in2/1 -> pfb_fir_1/1(pol1_in)
  pfb_fir_1/1(pol1_out) -> out2/1
  in3/1 -> pfb_fir_1/2(pol2_in)
  pfb_fir_1/2(pol2_out) -> out3/1
  sync_in/1 -> pfb_fir_1/3(sync_in), pfb_fir_0/3(sync_in)
  pfb_fir_0/3(sync_out) -> Terminator/1
  pfb_fir_1/3(sync_out) -> sync_out/1

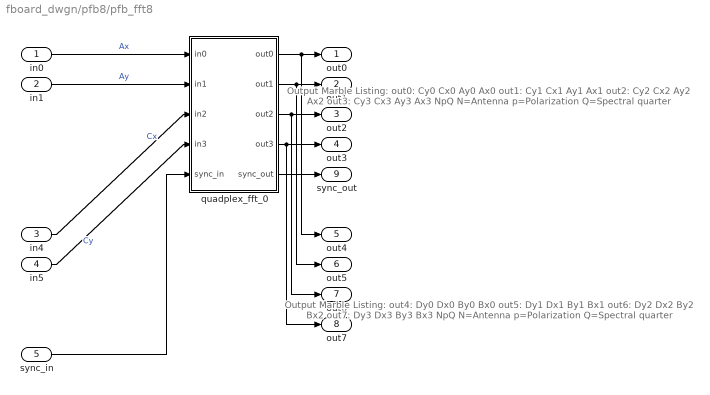
== system fboard_dwgn/pfb8/pfb_fft8 ==
  note: Output Marble Listing:
      |
      | out0: Cy0 Cx0 Ay0 Ax0
      | out1: Cy1 Cx1 Ay1 Ax1
      | out2: Cy2 Cx2 Ay2 Ax2
      | out3: Cy3 Cx3 Ay3 Ax3
      |
      | NpQ
      | N=Antenna
      | p=Polarization
      | Q=Spectral quarter
  note: Output Marble Listing:
      |
      | out4: Dy0 Dx0 By0 Bx0
      | out5: Dy1 Dx1 By1 Bx1
      | out6: Dy2 Dx2 By2 Bx2
      | out7: Dy3 Dx3 By3 Bx3
      |
      | NpQ
      | N=Antenna
      | p=Polarization
      | Q=Spectral quarter
  in0 : Inport  Port=1  LatchInput=off
  in1 : Inport  Port=2  LatchInput=off
  in4 : Inport  Port=3  LatchInput=off
  in5 : Inport  Port=4  LatchInput=off
  sync_in : Inport  Port=5  LatchInput=off
  quadplex_fft_0 : Subsystem
  out0 : Outport
  out1 : Outport  Port=2
  out2 : Outport  Port=3
  out3 : Outport  Port=4
  out4 : Outport  Port=5
  out5 : Outport  Port=6
  out6 : Outport  Port=7
  out7 : Outport  Port=8
  sync_out : Outport  Port=9
  wires:
  in0/1 -> quadplex_fft_0/1(in0)  "Ax"
  quadplex_fft_0/1(out0) -> out0/1, out4/1
  in1/1 -> quadplex_fft_0/2(in1)  "Ay"
  quadplex_fft_0/2(out1) -> out1/1, out5/1
  quadplex_fft_0/3(out2) -> out2/1, out6/1
  quadplex_fft_0/4(out3) -> out3/1, out7/1
  sync_in/1 -> quadplex_fft_0/5(sync_in)
  quadplex_fft_0/5(sync_out) -> sync_out/1
  in4/1 -> quadplex_fft_0/3(in2)  "Cx"
  in5/1 -> quadplex_fft_0/4(in3)  "Cy"

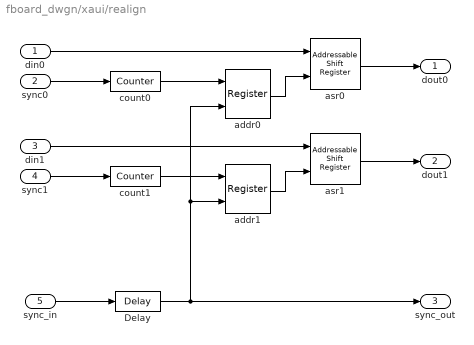
== system fboard_dwgn/xaui/realign ==
  din0 : Inport  Port=1  LatchInput=off
  sync0 : Inport  Port=2  LatchInput=off
  din1 : Inport  Port=3  LatchInput=off
  sync1 : Inport  Port=4  LatchInput=off
  sync_in : Inport  Port=5  LatchInput=off
  Delay : xbsIndex_r3/Delay  latency=1  reg_retiming=off  explicit_period=off  period=1  en=off  accept_only_valid=off  init_zero=on  dbl_ovrd=off  show_param=off
      settings: xl_area=[1 1 0 0 0 0 0]
  addr0 : xbsIndex_r3/Register  init=0  reg_only_valid=off  explicit_period=off  period=1  rst=off  en=on  out_en=off  dbl_ovrd=off  show_param=on
      settings: xl_area=[3 6 0 0 0 0 0]
  addr1 : xbsIndex_r3/Register  init=0  reg_only_valid=off  explicit_period=off  period=1  rst=off  en=on  out_en=off  dbl_ovrd=off  show_param=on
      settings: xl_area=[3 6 0 0 0 0 0]
  asr0 : xbsIndex_r3/Addressable Shift Register  infer_latency=on  depth=2  initVector=[0]  explicit_period=off  period=1  accept_only_valid=off  en=off  dbl_ovrd=off  show_param=on  use_rpm=on  gen_core=off
      settings: xl_area=[192 0 0 384 0 0 0]
  asr1 : xbsIndex_r3/Addressable Shift Register  infer_latency=on  depth=2  initVector=[0]  explicit_period=off  period=1  accept_only_valid=off  en=off  dbl_ovrd=off  show_param=on  use_rpm=on  gen_core=off
      settings: xl_area=[192 0 0 384 0 0 0]
  count0 : xbsIndex_r3/Counter  cnt_type=Free Running  n_bits=6  bin_pt=0  arith_type=Unsigned  start_count=0  cnt_to=Inf  cnt_by_val=1  operation=Up  explicit_period=off  period=1  load_pin=off  rst=on  en=off  dbl_ovrd=off  show_param=on  use_rpm=on  gen_core=off
      settings: xl_area=[3 6 0 6 0 0 0]
  count1 : xbsIndex_r3/Counter  cnt_type=Free Running  n_bits=6  bin_pt=0  arith_type=Unsigned  start_count=0  cnt_to=Inf  cnt_by_val=1  operation=Up  explicit_period=off  period=1  load_pin=off  rst=on  en=off  dbl_ovrd=off  show_param=on  use_rpm=on  gen_core=off
      settings: xl_area=[3 6 0 6 0 0 0]
  dout0 : Outport
  dout1 : Outport  Port=2
  sync_out : Outport  Port=3
  wires:
  count0/1 -> addr0/1
  addr0/1 -> asr0/2
  count1/1 -> addr1/1
  addr1/1 -> asr1/2
  Delay/1 -> addr1/2, addr0/2, sync_out/1
  din0/1 -> asr0/1
  asr0/1 -> dout0/1
  sync0/1 -> count0/1
  din1/1 -> asr1/1
  asr1/1 -> dout1/1
  sync1/1 -> count1/1
  sync_in/1 -> Delay/1

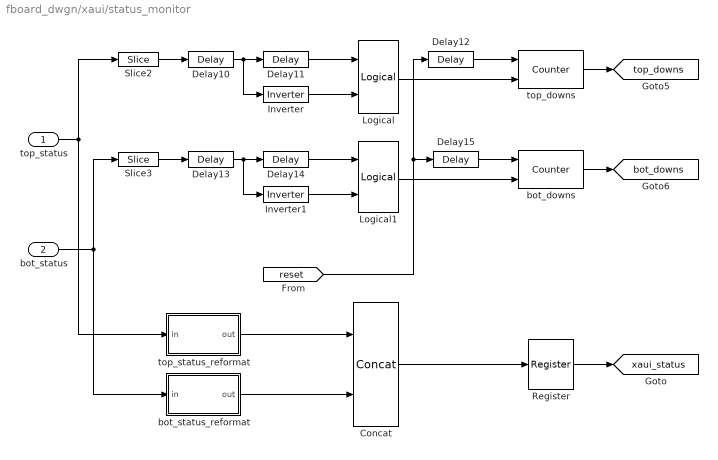
== system fboard_dwgn/xaui/status_monitor ==
  top_status : Inport  Port=1  LatchInput=off
  bot_status : Inport  Port=2  LatchInput=off
  Concat : xbsIndex_r3/Concat  num_inputs=2  explicit_period=off  period=1  dbl_ovrd=off
  Delay{10..15} (6 alike) : xbsIndex_r3/Delay  latency=1  reg_retiming=off  explicit_period=off  period=1  en=off  accept_only_valid=off  init_zero=on  dbl_ovrd=off  show_param=off
      settings: xl_area=[0, 0, 0, 0, 0, 0, 0]
  Inverter : xbsIndex_r3/Inverter  latency=0  explicit_period=off  period=1  en=off  dbl_ovrd=off  show_param=off
      settings: xl_area=[0, 0, 0, 0, 0, 0, 0]
  Inverter1 : xbsIndex_r3/Inverter  latency=0  explicit_period=off  period=1  en=off  dbl_ovrd=off  show_param=off
      settings: xl_area=[0, 0, 0, 0, 0, 0, 0]
  Logical : xbsIndex_r3/Logical  logical_function=AND  inputs=2  precision=Full  arith_type=Unsigned  n_bits=8  bin_pt=2  align_bp=on  latency=0  explicit_period=off  period=1  en=off  dbl_ovrd=off  show_param=off
      settings: xl_area=[0, 0, 0, 0, 0, 0, 0]
  Logical1 : xbsIndex_r3/Logical  logical_function=AND  inputs=2  precision=Full  arith_type=Unsigned  n_bits=8  bin_pt=2  align_bp=on  latency=0  explicit_period=off  period=1  en=off  dbl_ovrd=off  show_param=off
      settings: xl_area=[0, 0, 0, 0, 0, 0, 0]
  Register : xbsIndex_r3/Register  init=0  reg_only_valid=off  explicit_period=off  period=1  rst=off  en=off  out_en=off  dbl_ovrd=off  show_param=off
      settings: xl_area=[0, 0, 0, 0, 0, 0, 0]
  Slice2 : xbsIndex_r3/Slice  mode=Lower Bit Location + Width  nbits=1  bit1=12  base1=MSB of Input  bit0=12  base0=LSB of Input  boolean_output=on  explicit_period=off  period=1  dbl_ovrd=off
  Slice3 : xbsIndex_r3/Slice  mode=Lower Bit Location + Width  nbits=1  bit1=12  base1=MSB of Input  bit0=12  base0=LSB of Input  boolean_output=on  explicit_period=off  period=1  dbl_ovrd=off
  bot_downs : xbsIndex_r3/Counter  cnt_type=Free Running  n_bits=32  bin_pt=0  arith_type=Unsigned  start_count=0  cnt_to=Inf  cnt_by_val=1  operation=Up  explicit_period=off  period=1  load_pin=off  rst=on  en=on  dbl_ovrd=off  show_param=off  use_rpm=on  gen_core=off
      settings: xl_area=[0, 0, 0, 0, 0, 0, 0]
  bot_status_reformat : Subsystem
  top_downs : xbsIndex_r3/Counter  cnt_type=Free Running  n_bits=32  bin_pt=0  arith_type=Unsigned  start_count=0  cnt_to=Inf  cnt_by_val=1  operation=Up  explicit_period=off  period=1  load_pin=off  rst=on  en=on  dbl_ovrd=off  show_param=off  use_rpm=on  gen_core=off
      settings: xl_area=[0, 0, 0, 0, 0, 0, 0]
  top_status_reformat : Subsystem
  tag scope: bot_downs=global, top_downs=global, xaui_status=global
  wires:
  [reset] -> Delay15/1, Delay12/1
  Delay10/1 -> Delay11/1, Inverter/1
  Delay11/1 -> Logical/1
  Inverter/1 -> Logical/2
  Delay12/1 -> top_downs/1
  top_downs/1 -> [top_downs]
  Delay13/1 -> Delay14/1, Inverter1/1
  Delay14/1 -> Logical1/1
  Inverter1/1 -> Logical1/2
  Delay15/1 -> bot_downs/1
  bot_downs/1 -> [bot_downs]
  Logical1/1 -> bot_downs/2
  Logical/1 -> top_downs/2
  top_status/1 -> Slice2/1, top_status_reformat/1(in)
  bot_status/1 -> Slice3/1, bot_status_reformat/1(in)
  Slice2/1 -> Delay10/1
  Slice3/1 -> Delay13/1
  top_status_reformat/1(out) -> Concat/1
  bot_status_reformat/1(out) -> Concat/2
  Register/1 -> [xaui_status]
  Concat/1 -> Register/1

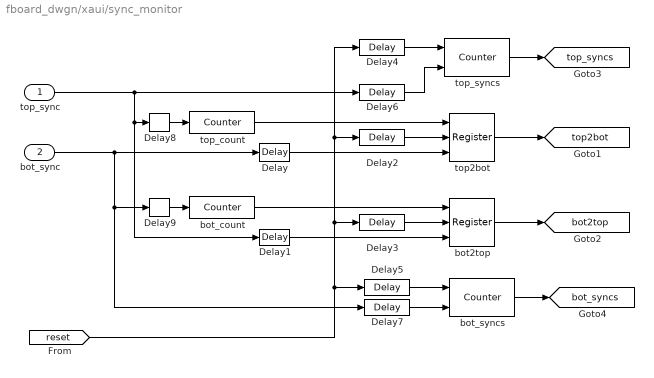
== system fboard_dwgn/xaui/sync_monitor ==
  top_sync : Inport  Port=1  LatchInput=off
  bot_sync : Inport  Port=2  LatchInput=off
  Delay : xbsIndex_r3/Delay  latency=2  reg_retiming=off  explicit_period=off  period=1  en=off  accept_only_valid=off  init_zero=on  dbl_ovrd=off  show_param=off
      settings: xl_area=[0, 0, 0, 0, 0, 0, 0]
  Delay1 : xbsIndex_r3/Delay  latency=2  reg_retiming=off  explicit_period=off  period=1  en=off  accept_only_valid=off  init_zero=on  dbl_ovrd=off  show_param=off
      settings: xl_area=[0, 0, 0, 0, 0, 0, 0]
  Delay{2..9} (8 alike) : xbsIndex_r3/Delay  latency=1  reg_retiming=off  explicit_period=off  period=1  en=off  accept_only_valid=off  init_zero=on  dbl_ovrd=off  show_param=off
      settings: xl_area=[0, 0, 0, 0, 0, 0, 0]
  bot2top : xbsIndex_r3/Register  init=hex2dec('ffffffff')  reg_only_valid=off  explicit_period=off  period=1  rst=on  en=on  out_en=off  dbl_ovrd=off  show_param=off
      settings: xl_area=[0, 0, 0, 0, 0, 0, 0]
  bot_count : xbsIndex_r3/Counter  cnt_type=Free Running  n_bits=32  bin_pt=0  arith_type=Unsigned  start_count=0  cnt_to=Inf  cnt_by_val=1  operation=Up  explicit_period=off  period=1  load_pin=off  rst=on  en=off  dbl_ovrd=off  show_param=off  use_rpm=on  gen_core=off
      settings: xl_area=[0, 0, 0, 0, 0, 0, 0]
  bot_syncs : xbsIndex_r3/Counter  cnt_type=Free Running  n_bits=32  bin_pt=0  arith_type=Unsigned  start_count=0  cnt_to=Inf  cnt_by_val=1  operation=Up  explicit_period=off  period=1  load_pin=off  rst=on  en=on  dbl_ovrd=off  show_param=off  use_rpm=on  gen_core=off
      settings: xl_area=[0, 0, 0, 0, 0, 0, 0]
  top2bot : xbsIndex_r3/Register  init=hex2dec('ffffffff')  reg_only_valid=off  explicit_period=off  period=1  rst=on  en=on  out_en=off  dbl_ovrd=off  show_param=off
      settings: xl_area=[0, 0, 0, 0, 0, 0, 0]
  top_count : xbsIndex_r3/Counter  cnt_type=Free Running  n_bits=32  bin_pt=0  arith_type=Unsigned  start_count=0  cnt_to=Inf  cnt_by_val=1  operation=Up  explicit_period=off  period=1  load_pin=off  rst=on  en=off  dbl_ovrd=off  show_param=off  use_rpm=on  gen_core=off
      settings: xl_area=[0, 0, 0, 0, 0, 0, 0]
  top_syncs : xbsIndex_r3/Counter  cnt_type=Free Running  n_bits=32  bin_pt=0  arith_type=Unsigned  start_count=0  cnt_to=Inf  cnt_by_val=1  operation=Up  explicit_period=off  period=1  load_pin=off  rst=on  en=on  dbl_ovrd=off  show_param=off  use_rpm=on  gen_core=off
      settings: xl_area=[0, 0, 0, 0, 0, 0, 0]
  tag scope: bot2top=global, bot_syncs=global, top2bot=global, top_syncs=global
  wires:
  bot_sync/1 -> Delay9/1, Delay7/1, Delay/1
  top_count/1 -> top2bot/1
  bot_count/1 -> bot2top/1
  Delay/1 -> top2bot/3
  Delay1/1 -> bot2top/3
  Delay2/1 -> top2bot/2
  Delay3/1 -> bot2top/2
  top2bot/1 -> [top2bot]
  bot2top/1 -> [bot2top]
  Delay4/1 -> top_syncs/1
  Delay5/1 -> bot_syncs/1
  top_syncs/1 -> [top_syncs]
  bot_syncs/1 -> [bot_syncs]
  Delay6/1 -> top_syncs/2
  Delay7/1 -> bot_syncs/2
  Delay8/1 -> top_count/1
  Delay9/1 -> bot_count/1
  top_sync/1 -> Delay1/1, Delay8/1, Delay6/1
  [reset] -> Delay3/1, Delay2/1, Delay4/1, Delay5/1

== system fboard_dwgn/xaui/sync_sel ==
  top_sync : Inport  Port=1  LatchInput=off
  bot_sync : Inport  Port=2  LatchInput=off
  Delay : xbsIndex_r3/Delay  latency=32  reg_retiming=off  explicit_period=off  period=1  en=off  accept_only_valid=off  init_zero=on  dbl_ovrd=off  show_param=off
      settings: xl_area=[0, 0, 0, 0, 0, 0, 0]
  Mux : xbsIndex_r3/Mux  inputs=2  precision=Full  arith_type="Signed  (2's comp)"  n_bits=8  bin_pt=2  quantization=Truncate  overflow=Wrap  latency=0  explicit_period=off  period=1  en=off  dbl_ovrd=off  show_param=off  mux_type=off  use_rpm=off  gen_core=off
      settings: xl_area=[0, 0, 0, 0, 0, 0, 0]
  bit0 : xbsIndex_r3/Slice  mode=Lower Bit Location + Width  nbits=1  bit1=12  base1=MSB of Input  bit0=12  base0=LSB of Input  boolean_output=on  explicit_period=off  period=1  dbl_ovrd=off
  sync_out : Outport
  wires:
  Mux/1 -> Delay/1
  top_sync/1 -> Mux/2
  bot_sync/1 -> Mux/3
  Delay/1 -> sync_out/1
  bit0/1 -> Mux/1
  [reg0] -> bit0/1

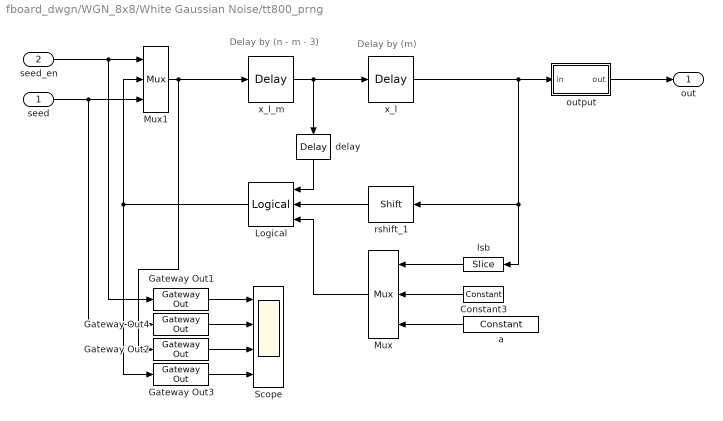
== system fboard_dwgn/WGN_8x8/White Gaussian Noise/tt800_prng ==
  note: Delay by (n - m - 3)
  note: Delay by (m)
  seed : Inport  Port=1  LatchInput=off
  seed_en : Inport  Port=2  LatchInput=off
  Constant3 : xbsIndex_r3/Constant  Orientation=left  const=0  equ=P=C  arith_type=Unsigned  n_bits=32  bin_pt=0  opselect=C  inp2=PCIN>>17  opr=+  inp1=P  carry=CIN  iostate=0  explicit_period=off  period=1  dbl_ovrd=off
  Gateway Out{1..4} (4 alike) : xbsIndex_r3/Gateway Out  output_type=Double  nbits=8  bin_pt=6  arith_type=Boolean  quantization=Truncate  overflow=Wrap  hdl_port=off  timing_constraint=None  locs_specified=off  LOCs={}  needs_fixed_name=off  show_param=off
      settings: xl_area=[0 0 0 0 0 0 0]
  Logical : xbsIndex_r3/Logical  Orientation=left  logical_function=XOR  inputs=3  precision=Full  arith_type=Unsigned  n_bits=8  bin_pt=2  align_bp=off  latency=1  explicit_period=off  period=1  en=off  dbl_ovrd=off  show_param=on
      settings: xl_area=[32 32 0 32 0 0 0]
  Mux : xbsIndex_r3/Mux  Orientation=left  inputs=2  precision=Full  arith_type="Signed  (2's comp)"  n_bits=8  bin_pt=2  quantization=Truncate  overflow=Wrap  latency=1  explicit_period=off  period=1  en=off  dbl_ovrd=off  show_param=off  mux_type=off  use_rpm=off  gen_core=off
      settings: xl_area=[16 32 0 32 0 0 0]
  Mux1 : xbsIndex_r3/Mux  inputs=2  precision=Full  arith_type="Signed  (2's comp)"  n_bits=8  bin_pt=2  quantization=Truncate  overflow=Wrap  latency=1  explicit_period=on  period=1  en=off  dbl_ovrd=off  show_param=on  mux_type=off  use_rpm=off  gen_core=off
      settings: xl_area=[16 32 0 32 0 0 0]
  Scope : Scope  NumInputPorts=4
      settings: YMin=-5~-5~-5~-5  YMax=5~5~5~5
  a : xbsIndex_r3/Constant  Orientation=left  const=hex2dec('8EBFD028')  equ=P=C  arith_type=Unsigned  n_bits=32  bin_pt=0  opselect=C  inp2=PCIN>>17  opr=+  inp1=P  carry=CIN  iostate=0  explicit_period=off  period=1  dbl_ovrd=off
  delay : xbsIndex_r3/Delay  Orientation=down  latency=1  reg_retiming=off  explicit_period=off  period=1  en=off  accept_only_valid=off  init_zero=on  dbl_ovrd=off  show_param=off
      settings: xl_area=[16 32 0 0 0 0 0]
  lsb : xbsIndex_r3/Slice  Orientation=left  mode=Lower Bit Location + Width  nbits=1  bit1=0  base1=MSB of Input  bit0=0  base0=LSB of Input  boolean_output=off  explicit_period=off  period=1  dbl_ovrd=off
  output : Subsystem
  rshift_1 : xbsIndex_r3/Shift  Orientation=left  shift_dir=Right  shift_bits=1  precision=User Defined  arith_type=Unsigned  n_bits=32  bin_pt=0  quantization=Truncate  overflow=Wrap  latency=1  explicit_period=off  period=1  en=off  dbl_ovrd=off  show_param=off
      settings: xl_area=[0 32 0 0 0 0 0]
  x_l : xbsIndex_r3/Delay  latency=7  reg_retiming=off  explicit_period=off  period=1  en=off  accept_only_valid=off  init_zero=on  dbl_ovrd=off  show_param=off
      settings: xl_area=[16 32 0 32 0 0 0]
  x_l_m : xbsIndex_r3/Delay  latency=25-7-3  reg_retiming=off  explicit_period=off  period=1  en=off  accept_only_valid=off  init_zero=on  dbl_ovrd=off  show_param=off
      settings: xl_area=[16 32 0 32 0 0 0]
  out : Outport
  wires:
  delay/1 -> Logical/1
  output/1(out) -> out/1
  Gateway Out3/1 -> Scope/4
  Gateway Out2/1 -> Scope/3
  Gateway Out4/1 -> Scope/2
  Gateway Out1/1 -> Scope/1
  seed/1 -> Mux1/3, Gateway Out4/1
  seed_en/1 -> Mux1/1, Gateway Out1/1
  Mux1/1 -> Gateway Out2/1, x_l_m/1
  Logical/1 -> Mux1/2, Gateway Out3/1
  Mux/1 -> Logical/3
  rshift_1/1 -> Logical/2
  a/1 -> Mux/3
  Constant3/1 -> Mux/2
  lsb/1 -> Mux/1
  x_l/1 -> output/1(in), rshift_1/1, lsb/1
  x_l_m/1 -> delay/1, x_l/1

== system fboard_dwgn/WGN_8x8/White Gaussian Noise/tt800_seed_gen ==
  seed_in : Inport  Port=1  LatchInput=off
  ld : Inport  Port=2  LatchInput=off
  Expression : xbsIndex_r3/Expression  expression=ld | ld_ext  precision=Full  arith_type=Unsigned  n_bits=8  bin_pt=2  align_bp=on  latency=1  explicit_period=off  period=1  en=off  dbl_ovrd=off  show_param=on
      settings: xl_area=[0, 0, 0, 0, 0, 0, 0]
  LFSR : xbsIndex_r3/LFSR  lfsr_type=Fibonacci  gate_type=XOR  output_type=on  n_bits=32  bin_pt=0  arith_type=Unsigned  polynomial='C0000401'  rst_value=dec2hex(seed)  reloadable_seed=on  input_type=on  explicit_period=on  period=1  rst=off  en=off  dbl_ovrd=off  show_param=on  useSRL16s=off  use_rpm=off  gen_core=off
      settings: xl_area=[17 32 0 33 0 0 0]
  p24_extender : Subsystem
  r_edge_detect : Subsystem
  seed_out : Outport
  seed_en : Outport  Port=2
  wires:
  r_edge_detect/1(out) -> p24_extender/1(in)
  p24_extender/1(out) -> Expression/2
  ld/1 -> LFSR/2, r_edge_detect/1(in), Expression/1
  Expression/1 -> seed_en/1
  seed_in/1 -> LFSR/1
  LFSR/1 -> seed_out/1

== system fboard_dwgn/WGN_8x8/White Gaussian Noise/u2n ==
  u : Inport  Port=1  LatchInput=off
  Gateway Out : xbsIndex_r3/Gateway Out  output_type=Double  nbits=8  bin_pt=6  arith_type=Boolean  quantization=Truncate  overflow=Wrap  hdl_port=off  timing_constraint=None  locs_specified=off  LOCs={}  needs_fixed_name=off  show_param=off
      settings: xl_area=[0 0 0 0 17 0 0]
  Gateway Out1 : xbsIndex_r3/Gateway Out  output_type=Double  nbits=8  bin_pt=6  arith_type=Boolean  quantization=Truncate  overflow=Wrap  hdl_port=off  timing_constraint=None  locs_specified=off  LOCs={}  needs_fixed_name=off  show_param=off
      settings: xl_area=[0 0 0 0 17 0 0]
  Scope : Scope  NumInputPorts=2
      settings: YMin=-5~-5  YMax=5~5
  SineCosine : xbsIndex_r3/SineCosine  mode=Sine and Cosine  neg_sin=off  neg_cos=off  n_bits=8  latency=2  sym_output=off  explicit_period=off  period=1  en=off  dbl_ovrd=off  show_param=on  mem_type=Block RAM  pipeline=on  use_rpm=on  gen_core=off
      settings: xl_area=[8 16 1 2 0 0 0]
  bottom_11 : xbsIndex_r3/Slice  mode=Lower Bit Location + Width  nbits=11  bit1=0  base1=MSB of Input  bit0=0  base0=LSB of Input  boolean_output=off  explicit_period=off  period=1  dbl_ovrd=off
  log_lut : xbsIndex_r3/ROM  depth=2^11  initVector=quant(sqrt(-2*log(linspace(2^-11,1,2^11))),2^-7)  arith_type=Unsigned  n_bits=9  bin_pt=7  latency=1  init_zero=on  explicit_period=off  period=1  rst=off  init_reg=0  en=off  dbl_ovrd=off  show_param=off  distributed_mem=off  use_rpm=off  gen_core=off
      settings: xl_area=[0 0 1 0 0 0 0]
  r_cos : xbsIndex_r3/Mult  precision=Full  arith_type="Signed  (2's comp)"  n_bits=8  bin_pt=2  quantization=Truncate  overflow=Wrap  latency=3  explicit_period=off  period=1  en=off  dbl_ovrd=off  show_param=on  mult_type=Parallel  oversample=2  use_embedded=on  pipeline=on  use_rpm=on  placement_style=Rectangular Shape  gen_core=off
      settings: xl_area=[18 34 0 17 0 1 0]
  r_sin : xbsIndex_r3/Mult  precision=Full  arith_type="Signed  (2's comp)"  n_bits=8  bin_pt=2  quantization=Truncate  overflow=Wrap  latency=3  explicit_period=off  period=1  en=off  dbl_ovrd=off  show_param=on  mult_type=Parallel  oversample=2  use_embedded=on  pipeline=on  use_rpm=on  placement_style=Rectangular Shape  gen_core=off
      settings: xl_area=[18 34 0 17 0 1 0]
  top_11 : xbsIndex_r3/Slice  mode=Upper Bit Location + Width  nbits=11  bit1=0  base1=MSB of Input  bit0=0  base0=MSB of Input  boolean_output=off  explicit_period=off  period=1  dbl_ovrd=off
  n1 : Outport
  n2 : Outport  Port=2
  wires:
  Gateway Out/1 -> Scope/1
  Gateway Out1/1 -> Scope/2
  bottom_11/1 -> SineCosine/1
  top_11/1 -> log_lut/1
  u/1 -> top_11/1, bottom_11/1
  SineCosine/2 -> r_cos/2
  log_lut/1 -> r_sin/1, r_cos/1
  SineCosine/1 -> r_sin/2
  r_sin/1 -> Gateway Out/1, n1/1
  r_cos/1 -> Gateway Out1/1, n2/1
